simulink model "test_pwm"  (R2020b)
settings: Solver=FixedStepAuto  StartTime=0.0  StopTime=100  RelTol=1e-3  EnableMultiTasking=on
undefined symbols (not defined in the file or in its folder): DiscIntNeverNeededParam
libraries: simulink x5
settings Model: EnablePacing=on  ExtModeTrigDuration=100  Creator=Zein  LastModifiedBy=Zein
settings SolverCC: PositivePriorityOrder=on
settings OptimizationCC: DefaultParameterBehavior=Inlined  EnhancedBackFolding=on  PassReuseOutputArgsAs=Individual arguments  ZeroExternalMemoryAtStartup=off  ZeroInternalMemoryAtStartup=off  MaxStackSize=64  OptimizeBlockOrder=speed  DifferentSizesBufferReuse=on  OptimizationCustomize=off  EfficientTunableParamExpr=on
settings DebuggingCC: ParameterTunabilityLossMsg=error
settings HardwareCC: ProdBitPerPointer=32  ProdBitPerSizeT=32  ProdBitPerPtrDiffT=32  ProdLargestAtomicInteger=Long  ProdLargestAtomicFloat=Double  ProdWordSize=32  ProdHWDeviceType=ARM Compatible->ARM Cortex
settings SFSimCC: MATLABDynamicMemAlloc=off
settings RTWCC: Description=Embedded Coder  SystemTargetFile=ert.tlc  TemplateMakefile=ert_default_tmf  Toolchain=GNU GCC BeagleBone Blue
settings CodeAppCC: ForceParamTrailComments=on  IgnoreCustomStorageClasses=off  OperatorAnnotations=on  SimulinkDataObjDesc=on  SFDataObjDesc=on  InsertBlockDesc=on
settings ERTTargetCC: SupportVariableSizeSignals=on  ERTCustomFileTemplate=example_file_process.tlc

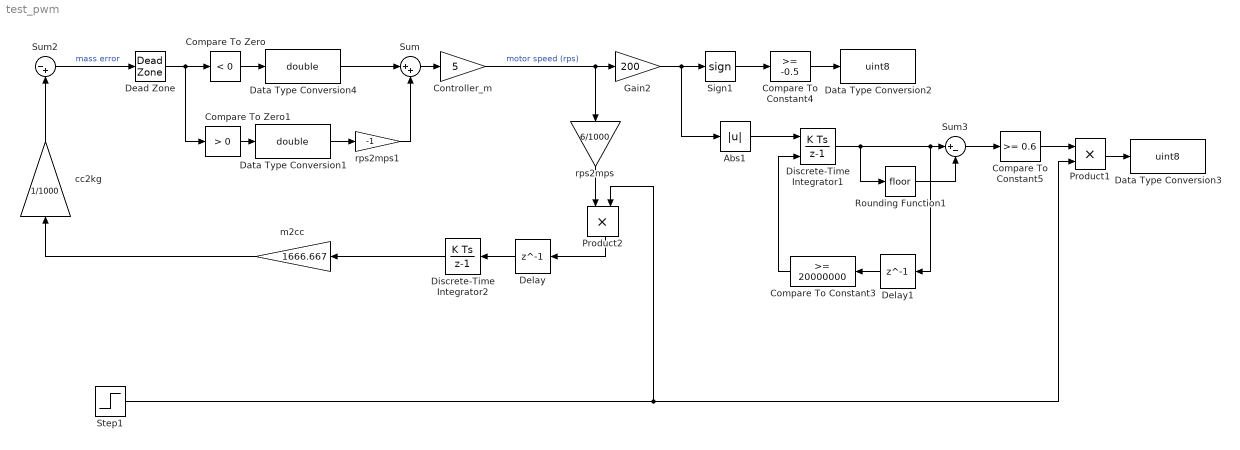
== system test_pwm ==
  Abs1 : Abs
  Compare To Constant3 : simulink/Logic and Bit Operations/Compare To Constant  relop=>=  const=20000000  OutDataTypeStr=boolean
  Compare To Constant4 : simulink/Logic and Bit Operations/Compare To Constant  relop=>=  const=-0.5  OutDataTypeStr=boolean
  Compare To Constant5 : simulink/Logic and Bit Operations/Compare To Constant  relop=>=  const=0.6  OutDataTypeStr=uint8
  Compare To Zero : simulink/Logic and Bit Operations/Compare To Zero  relop=<  OutDataTypeStr=boolean
  Compare To Zero1 : simulink/Logic and Bit Operations/Compare To Zero  relop=>  OutDataTypeStr=boolean
  Controller_m : Gain  Gain=5
  Data Type Conversion1 : DataTypeConversion  OutDataTypeStr=double
  Data Type Conversion2 : DataTypeConversion  OutDataTypeStr=uint8
  Data Type Conversion3 : DataTypeConversion  OutDataTypeStr=uint8
  Data Type Conversion4 : DataTypeConversion  OutDataTypeStr=double
  Dead Zone : DeadZone  LowerValue=-0.0001  UpperValue=0.0001  SaturateOnIntegerOverflow=on
  Delay : Delay  DelayLength=1  SampleTime=1/5000
  Delay1 : Delay  DelayLength=1
  Discrete-Time Integrator1 : DiscreteIntegrator  ExternalReset=rising  SampleTime=1/5000  ICPrevOutput=DiscIntNeverNeededParam  ICPrevScaledInput=DiscIntNeverNeededParam
  Discrete-Time Integrator2 : DiscreteIntegrator  SampleTime=1/5000  ICPrevOutput=DiscIntNeverNeededParam  ICPrevScaledInput=DiscIntNeverNeededParam
  Gain2 : Gain  Gain=200
  Product1 : Product
  Product2 : Product
  Rounding Function1 : Rounding
  Sign1 : Signum
  Step1 : Step  Time=3
  Sum : Sum  Inputs=|++
  Sum2 : Sum  Inputs=|-+
  Sum3 : Sum  Inputs=|+-
  cc2kg : Gain  Gain=1/1000
  m2cc : Gain  Gain=1666.667
  rps2mps : Gain  Gain=6/1000
  rps2mps1 : Gain  Gain=-1
  wires:
  Sum2/1 -> Dead Zone/1  "mass error"
  Discrete-Time Integrator2/1 -> m2cc/1
  m2cc/1 -> cc2kg/1
  Delay/1 -> Discrete-Time Integrator2/1
  Abs1/1 -> Discrete-Time Integrator1/1
  Controller_m/1 -> rps2mps/1, Gain2/1  "motor speed (rps)"
  Gain2/1 -> Abs1/1, Sign1/1
  Compare To Constant5/1 -> Product1/1
  rps2mps/1 -> Product2/1
  Sign1/1 -> Compare To Constant4/1
  Rounding Function1/1 -> Sum3/2
  Step1/1 -> Product1/2, Product2/2
  Discrete-Time Integrator1/1 -> Delay1/1, Sum3/1, Rounding Function1/1
  Compare To Constant3/1 -> Discrete-Time Integrator1/2
  Sum3/1 -> Compare To Constant5/1
  Delay1/1 -> Compare To Constant3/1
  Compare To Constant4/1 -> Data Type Conversion2/1
  Product1/1 -> Data Type Conversion3/1
  cc2kg/1 -> Sum2/2
  Dead Zone/1 -> Compare To Zero1/1, Compare To Zero/1
  Compare To Zero/1 -> Data Type Conversion4/1
  Compare To Zero1/1 -> Data Type Conversion1/1
  rps2mps1/1 -> Sum/2
  Sum/1 -> Controller_m/1
  Data Type Conversion4/1 -> Sum/1
  Data Type Conversion1/1 -> rps2mps1/1
  Product2/1 -> Delay/1
